simulink model "jetsonCart_nodeGen"  (R2020b)
settings: Solver=FixedStepAuto  StartTime=0.0  StopTime=inf  FixedStep=1/15  RelTol=1e-3
libraries: robotlib x6, simulink x1
settings Model: EnablePacing=on  Creator=iftach  LastModifiedBy=iftach
settings DataIOCC: ReturnWorkspaceOutputs=off
settings OptimizationCC: EnhancedBackFolding=on  PassReuseOutputArgsAs=Individual arguments  ZeroExternalMemoryAtStartup=off  ZeroInternalMemoryAtStartup=off  MaxStackSize=64  OptimizeBlockOrder=speed  DifferentSizesBufferReuse=on  OptimizationCustomize=off  EfficientTunableParamExpr=on
settings DebuggingCC: ParameterTunabilityLossMsg=error
settings HardwareCC: ProdBitPerLong=64  ProdHWDeviceType=Intel->x86-64 (Linux 64)
settings SFSimCC: MATLABDynamicMemAlloc=off  SimTargetLang=C++
settings RTWCC: Description=Embedded Coder  SystemTargetFile=ert.tlc  HardwareBoard=Robot Operating System (ROS)  TLCOptions="-aInlineSetEventsForThisBaseRateFcn=TLC_FALSE -aSuppressMultiTaskScheduler=TLC_FALSE  -aRateBasedStepFcn=0"  TemplateMakefile=ert_default_tmf  GenerateReport=on  Toolchain=Catkin  IncludeHyperlinkInReport=on  LaunchReport=on  TargetLang=C++  GenerateTraceInfo=on  GenerateTraceReport=on  GenerateTraceReportSl=on  GenerateTraceReportSf=on  GenerateTraceReportEml=on
settings CodeAppCC: ForceParamTrailComments=on  IgnoreCustomStorageClasses=off  OperatorAnnotations=on  SimulinkDataObjDesc=on  SFDataObjDesc=on  InsertBlockDesc=on
settings ERTTargetCC: SupportVariableSizeSignals=on

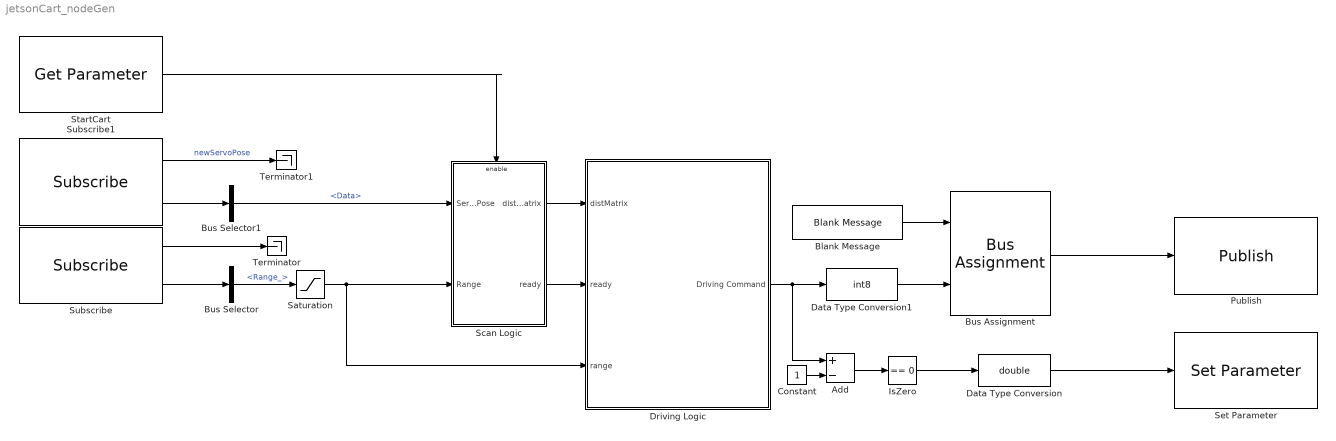
== system jetsonCart_nodeGen ==
  Add : Sum  Inputs=+-
  Blank Message : robotlib/Blank Message  messageClass=Message  entityType=std_msgs/Int8  messageType=std_msgs/Int8  SampleTime=inf  legacyBusStruct=off
  Bus Assignment : BusAssignment  AssignedSignals=Data
  Bus Selector : BusSelector  OutputSignals=Range_
  Bus Selector1 : BusSelector  OutputSignals=Data
  Constant : Constant
  Data Type Conversion : DataTypeConversion  OutDataTypeStr=double
  Data Type Conversion1 : DataTypeConversion  OutDataTypeStr=int8
  Driving Logic : Subsystem  TreatAsAtomicUnit=on
  IsZero : simulink/Logic and Bit Operations/Compare To Zero  relop===  OutDataTypeStr=boolean
  Publish : robotlib/Publish  topicSource=Specify your own  topic=/commands  messageType=std_msgs/Int8  legacyBusStruct=off  messageQueueLength=1
  Saturation : Saturate  UpperLimit=350  LowerLimit=0
  Scan Logic : Subsystem  TreatAsAtomicUnit=on
  Set Parameter : robotlib/Set Parameter  ParameterSource=Specify your own  ParameterName=/startCart  ParameterType=double  ModelName=jetsonCart_nodeGen  BlockId=ParamSet_jetsonCart_nodeGen_479
      settings: SourceProductBaseCode=RR
  StartCart : robotlib/Get Parameter  ParameterSource=Specify your own  ParameterName=/startCart  ParameterType=double  ParameterMaxArrayLength=16  ParameterInitialValue=0  SampleTime=-1  ShowErrorCodeOutput=off  ModelName=jetsonCart_nodeGen  BlockId=ParamGet_jetsonCart_nodeGen_471
      settings: SourceProductBaseCode=RR
  Subscribe : robotlib/Subscribe  topicSource=Specify your own  topic=/ultrasound  messageType=sensor_msgs/Range  SampleTime=-1  legacyBusStruct=off  messageQueueLength=1
  Subscribe1 : robotlib/Subscribe  topicSource=Specify your own  topic=/servo  messageType=std_msgs/UInt16  SampleTime=-1  legacyBusStruct=off  messageQueueLength=1
  Terminator : Terminator
  Terminator1 : Terminator
  wires:
  Subscribe/1 -> Terminator/1
  Subscribe/2 -> Bus Selector/1
  Subscribe1/2 -> Bus Selector1/1
  Bus Selector1/1 -> Scan Logic/1(ServoPose)  "<Data>"
  Bus Selector/1 -> Saturation/1  "<Range_>"
  Bus Assignment/1 -> Publish/1
  Blank Message/1 -> Bus Assignment/1
  Driving Logic/1(Driving Command) -> Add/1, Data Type Conversion1/1
  Scan Logic/2(ready) -> Driving Logic/2(ready)
  Scan Logic/1(distMatrix) -> Driving Logic/1(distMatrix)
  IsZero/1 -> Data Type Conversion/1
  Data Type Conversion/1 -> Set Parameter/1
  Data Type Conversion1/1 -> Bus Assignment/2
  Add/1 -> IsZero/1
  Constant/1 -> Add/2
  StartCart/1 -> Scan Logic/Enable
  Subscribe1/1 -> Terminator1/1  "newServoPose"
  Saturation/1 -> Driving Logic/3(range), Scan Logic/2(Range)

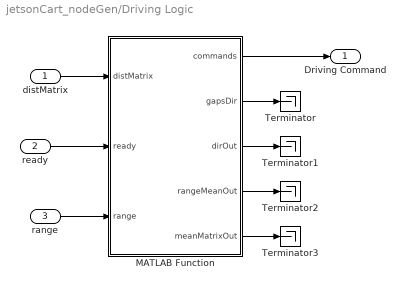
== system jetsonCart_nodeGen/Driving Logic ==
  distMatrix : Inport
  ready : Inport  Port=2
  range : Inport  Port=3
  MATLAB Function : MATLAB Function  TreatAsAtomicUnit=on
  Terminator{,1..3} (4 alike) : Terminator
  Driving Command : Outport
  wires:
  MATLAB Function/1(commands) -> Driving Command/1
  distMatrix/1 -> MATLAB Function/1(distMatrix)
  ready/1 -> MATLAB Function/2(ready)
  range/1 -> MATLAB Function/3(range)
  MATLAB Function/2(gapsDir) -> Terminator/1
  MATLAB Function/3(dirOut) -> Terminator1/1
  MATLAB Function/4(rangeMeanOut) -> Terminator2/1
  MATLAB Function/5(meanMatrixOut) -> Terminator3/1

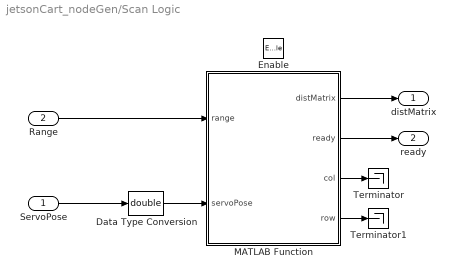
== system jetsonCart_nodeGen/Scan Logic ==
  ServoPose : Inport
  Range : Inport  Port=2
  Enable : EnablePort
  Data Type Conversion : DataTypeConversion  OutDataTypeStr=double
  MATLAB Function : MATLAB Function  TreatAsAtomicUnit=on
  Terminator : Terminator
  Terminator1 : Terminator
  distMatrix : Outport
  ready : Outport  Port=2
  wires:
  ServoPose/1 -> Data Type Conversion/1
  MATLAB Function/2(ready) -> ready/1
  MATLAB Function/1(distMatrix) -> distMatrix/1
  Data Type Conversion/1 -> MATLAB Function/2(servoPose)
  Range/1 -> MATLAB Function/1(range)
  MATLAB Function/3(col) -> Terminator/1
  MATLAB Function/4(row) -> Terminator1/1

== matlab function jetsonCart_nodeGen/Driving Logic/MATLAB Function ==
  data: distMatrix input; ready input; range input; commands output; gapsDir output; dirOut output; rangeMeanOut output; meanMatrixOut output
function [commands, gapsDir, dirOut, rangeMeanOut, meanMatrixOut]  = fcn(distMatrix, ready, range)%#codegen
persistent doneScanning counter matrixTmp cmdTmp gapsTmp dirTmp rangeTmp meanMatrixTmp

if isempty(matrixTmp)
    matrixTmp = zeros(4,51);
end
if isempty(meanMatrixTmp)
    meanMatrixTmp = zeros(1,51);
end
if isempty(gapsTmp)
    gapsTmp = zeros(1,51);
end
if isempty(rangeTmp)
    rangeTmp = 0;
end
if isempty(dirTmp)
    dirTmp = 0;
end
if isempty(counter)
    counter = 0;
end
if isempty(cmdTmp)
    cmdTmp = 0;
end


if isnan(ready)
    cmdTmp = 1;
    doneScanning = 0;
    counter = 0;
elseif ready == 0
    cmdTmp = 1;
    doneScanning = 0;
    counter = 0;
else
    doneScanning = 1;
    matrixTmp = distMatrix;
end

if doneScanning == 1 && counter == 0
    counter = 1;
    meanMatrix = mean(matrixTmp);
    meanMatrixTmp = meanMatrix;
    gaps = zeros(1,51);
    for i = 1 : length(meanMatrix) - 5
        gaps(i) = mean(meanMatrix(i:i+5));
    end
    gapsTmp = gaps;
    [RangeMean, dir] = max(gaps);
    dirTmp = dir;
    rangeTmp = RangeMean;
    if RangeMean < 50
        cmdTmp = 3;
    else
        if dir <= 30 && dir >= 15
            cmdTmp = 2;
        elseif dir > 30
            cmdTmp = 5;
        else 
            cmdTmp = 4;
        end
    end
end


gapsDir = gapsTmp;
dirOut = dirTmp;
rangeMeanOut = rangeTmp;
meanMatrixOut = meanMatrixTmp;

%servoDir = (dir/51)*100 + 36;

if range < 50 %emergency stop
    cmdTmp = 1;
end

if cmdTmp ~=1
    counter = counter +1;
end

%control
if cmdTmp == 2 || cmdTmp == 3 %driving time for backward or forward drive
    drivingTime = 60;%driving time for backward or forward drive
elseif cmdTmp == 4
    drivingTime = abs((1-15/dirOut)*10 + 10)/2;
else
    drivingTime = abs((1 - 30/dirOut)*60 + 10)/2;
end

if counter > drivingTime
    cmdTmp = 1;
    counter = 0;
end

commands = cmdTmp;

== matlab function jetsonCart_nodeGen/Scan Logic/MATLAB Function ==
  data: range input; distMatrix output; ready output; col output; row output; servoPose input
function [distMatrix, ready, col, row] = fcn(range, servoPose)%#codegen
persistent rangeMat i j flag

if isempty(rangeMat)
    rangeMat = zeros(4,51);
end

if isempty(i)
    i = 1;
end

if isempty(flag)
    flag = 0;
end

pose = servoPose;
if pose < 36
    pose = 36;
end
if pose > 136
    pose = 136;
end

if isempty(j)
    j = floor((pose - 36 + 2)/2);
end

if i < 5
    rangeMat(i,j) = range;
%     if flag == 1
%         j = j - 1;
%     else
%         j = j + 1;
%     end
    j = floor((pose - 36 + 2)/2);
end

if  j == 51 && flag == 0
    i = i+1;
    flag = 1;
end
if j == 1 && flag == 1
    flag = 0;
    i = i+1;
end

if  i == 5  
    ready = 1;
    i = 1;
    j = 1;
    flag = 0;
else
    ready = 0;
end

distMatrix = rangeMat;
col = j;
row = i;
